simulink model "lab8"  (R2019b)
settings: Solver=VariableStepAuto  StartTime=0.0  StopTime=100  RelTol=1e-3
settings Model: Creator=theojanson  LastModifiedBy=theojanson

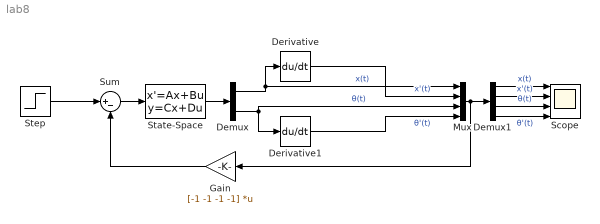
== system lab8 ==
  Demux : Demux  Outputs=2
  Demux1 : Demux
  Derivative : Derivative
  Derivative1 : Derivative
  Gain : Gain  Gain=[-1 -1 -1 -1]  Multiplication=Matrix(K*u) (u vector)
  Mux : Mux
  Scope : Scope  NumInputPorts=4
  State-Space : StateSpace  A=[0 1 0 0 ; 0 -14.4899 -1.9749 0 ; 0 0 0 1 ; 0 86.2495 58.3333 0]  B=[0 ; 3.255 ; 0 ; -19.3751]  C=[1 0 0 0 ; 0 0 1 0]  D=[0;0]  InitialCondition=[0 0 0.05 0]
  Step : Step  After=0  SampleTime=0
  Sum : Sum  Inputs=|+-
  wires:
  Demux/1 -> Mux/1, Derivative/1  "x(t)"
  Step/1 -> Sum/1
  Gain/1 -> Sum/2
  Demux/2 -> Derivative1/1, Mux/3  "θ(t)"
  State-Space/1 -> Demux/1
  Sum/1 -> State-Space/1
  Derivative/1 -> Mux/2  "x'(t)"
  Derivative1/1 -> Mux/4  "θ'(t)"
  Mux/1 -> Gain/1, Demux1/1
  Demux1/1 -> Scope/1  "x(t)"
  Demux1/2 -> Scope/2  "x'(t)"
  Demux1/3 -> Scope/3  "θ(t)"
  Demux1/4 -> Scope/4  "θ'(t)"
